simulink model "mech_interface_hyd_slidercrank"  (Simulink 7.1)
settings: Solver=ode15s  StartTime=0.0  StopTime=20  RelTol=1e-5
model workspace (MAT data in the model file):
  Lr = 0.5
  Lc = 0.288675134595
  sl_a = 0.5
  sl_b = 0.25
  sl_c = 0.25
  M_sl = 0.5
  I_sl = [0.0208333333333  0  0; 0  0.0520833333333  0; 0  0  0.0520833333333]
  rk_a = 0.5
  rk_b = 0.05
  rk_c = 0.05
  M_rk = 0.5
  I_rk = [0.000208333333333  0  0; 0  0.0105208333333  0; 0  0  0.0105208333333]
  cr_a = 0.288675
  cr_b = 0.05
  cr_c = 0.05
  M_cr = 5
  I_cr : num (value not decoded)
PostLoadFcn:
  | hws = get_param(bdroot, 'modelworkspace');
  | 
  | hws.assignin('sl_a', 0.5);
  | hws.assignin('sl_b', 0.25);
  | hws.assignin('sl_c', 0.25);
  | hws.assignin('M_sl', 0.5);
  | hws.evalin('I_sl = [1/3*M_sl*(sl_b^2 + sl_c^2) 0 0;   0 1/3*M_sl*(sl_a^2 + sl_c^2) 0;   0 0 1/3*M_sl*(sl_a^2 + sl_b^2)];')
  | 
  | hws.assignin('rk_a', 0.5);
  | hws.assignin('rk_b', 0.05);
  | hws.assignin('rk_c', 0.05);
  | hws.assignin('M_rk', 0.5);
  | hws.evalin('I_rk = [1/12*M_rk*(rk_b^2 + rk_c^2) 0 0;   0 1/12*M_rk*(rk_a^2 + rk_c^2) 0;   0 0 1/12*M_rk*(rk_a^2 + rk_b^2)];')
  | 
  | hws.assignin('cr_a', 0.288675);
  | hws.assignin('cr_b', 0.05);
  | hws.assignin('cr_c', 0.05);
  | hws.assignin('M_cr', 5);
  | hws.evalin('I_cr = [1/12*M_cr*(cr_b^2 + cr_c^2) 0 0;   0 1/12*M_cr*(cr_a^2 + cr_c^2) 0;   0 0 1/12*M_cr*(cr_a^2 + cr_b^2)];')
  | 
  | clear hws
undefined symbols (not defined in the file or in its folder): sigbuilder_block
libraries: mblibv1 x11, fl_lib x8, nesl_utility x3
Description:
  | Hydraulic - 3D Rotational Energy Conversion
  | 
  | The Rotational Hydraulic Actuator subsystem uses a Revolute-Rotational Interface block and Rotational Hydro-Mechanical Converter blocks to hydraulically actuate a revolute joint.
  | 
  | The hydraulic circuit is modeled in Simscape. The rest of the mechanism is modeled in SimMechanics.
settings Model: Creator=ksanthan  LastModifiedBy=batserve  ExtModeAutoUpdateStatusClock=off
settings SolverCC: SolverResetMethod=Robust
settings DataIOCC: SaveOutput=off  SignalLogging=off  SaveTime=off  OutputOption=SpecifiedOutputTimes  OutputTimes=[0:0.05:20]
settings DebuggingCC: AlgebraicLoopMsg=none  SignalResolutionControl=TryResolveAllWithWarning  SolverPrmCheckMsg=none
settings GRTTargetCC: TargetFcnLib=ansi_tfl_tmw_new.mat
settings SimMechanicsCC: VisOnUpdateDiagram=on  VisDuringSimulation=on

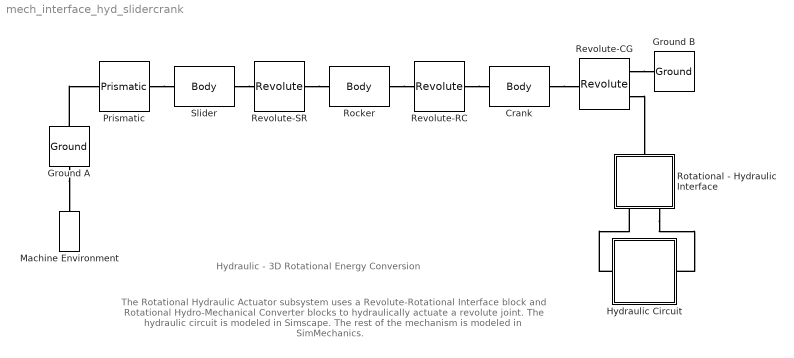
== system mech_interface_hyd_slidercrank ==
  note: Hydraulic - 3D Rotational Energy Conversion
  note: The Rotational Hydraulic Actuator subsystem uses a Revolute-Rotational Interface block and
      | Rotational Hydro-Mechanical Converter blocks to hydraulically actuate a revolute joint.
      |
      | The hydraulic circuit is modeled in Simscape.
      | The rest of the mechanism is modeled in SimMechanics.
  Crank : mblibv1/Bodies/Body  DialogController=MECH.DynMechDlgSource  PhysicalDomain=mechanical  SubClassName=Unknown  LeftPortType=workingframe  RightPortType=workingframe  LConnTagsString=CS1  RConnTagsString=CS2  DialogClass=MechanicalBodyBlock  Mass=M_cr  MassUnits=lbm  InertiaUnits=lbm*ft^2  Inertia=I_cr  Shape=Cylinder  ShapeDims=[1 1]  ShapeUnits=m  ShapeUse=false  Density=1  DensityUnits=kg/m^3  DensityUse=false  GraphicsMode=1  BodyColor=[0.5 0.5 0.5]  GraphicsObj=[]  AttachedToCS=1  CG=Left$CG$[cr_a 0 0]/2$CS1$CS1$ft$[0 0 0]$Euler X-Y-Z$deg$CS1$false  WorkingFrames=Left$CS1$[0 0 0]$Adjoining$Adjoining$ft$[0 0 -pi/2]$Euler X-Y-Z$rad$Adjoining$true#Right$CS2$[cr_a 0 0]$CS1$CS1$ft$[0 0 0]$Euler X-Y-Z$deg$CS1$true  CGPos=[cr_a 0 0]/2  CGRot=[0 0 0]  CS0Pos=[]  CS0Rot=[]  CS1Pos=[0 0 0]  CS1Rot=[0 0 -pi/2]  CS2Pos=[cr_a 0 0]  CS2Rot=[0 0 0]  CS3Pos=[]  CS3Rot=[]  CS4Pos=[]  CS4Rot=[]  CS5Pos=[]  CS5Rot=[]  CS6Pos=[]  CS6Rot=[]  CS7Pos=[]  CS7Rot=[]  CS8Pos=[]  CS8Rot=[]  CS9Pos=[]  CS9Rot=[]  CS10Pos=[]  CS10Rot=[]  CS11Pos=[]  CS11Rot=[]  CS12Pos=[]  CS12Rot=[]  CS13Pos=[]  CS13Rot=[]  CS14Pos=[]  CS14Rot=[]  CS15Pos=[]  CS15Rot=[]  CS16Pos=[]  CS16Rot=[]  CS17Pos=[]  CS17Rot=[]  CS18Pos=[]  CS18Rot=[]  CS19Pos=[]  CS19Rot=[]  CS20Pos=[]  CS20Rot=[]
  Ground A : mblibv1/Bodies/Ground  Orientation=up  DialogController=MECH.DynMechDlgSource  SystemSampleTime=-1  LeftPortType=env  RightPortType=workingframe  PhysicalDomain=Mechanical  DialogClass=GroundBlock  CoordPosition=[0 0 0]  CoordPositionUnits=m  StateVectorMgrId=-1  MachineId=[0 0]  ShowEnvPort=on
  Ground B : mblibv1/Bodies/Ground  Orientation=left  DialogController=MECH.DynMechDlgSource  SystemSampleTime=-1  LeftPortType=env  RightPortType=workingframe  PhysicalDomain=Mechanical  DialogClass=GroundBlock  CoordPosition=[Lr*cos(pi/6)+Lc*cos(pi/3)+1/24 0 0]  CoordPositionUnits=ft  StateVectorMgrId=-1  MachineId=[0 0]  ShowEnvPort=off
  Hydraulic Circuit : Subsystem
  Machine Environment : mblibv1/Bodies/Machine Environment  Tag=Factory ground  Orientation=up  DialogController=MECH.DialogSource  SystemSampleTime=-1  PortType=env  PhysicalDomain=Mechanical  DialogTemplateClass=MECH.MachineEnvironment  SyncWhenCopied=off  Gravity=[0 0 0]  GravityUnits=m/s^2  GravityAsSignal=off  Dimensionality=Auto-detect  AnalysisType=Forward dynamics  LinearAssemblyTolerance=1e-3  LinearAssemblyToleranceUnits=m  AngularAssemblyTolerance=1e-3  AngularAssemblyToleranceUnits=rad  ConstraintSolverType=Stabilizing  ConstraintRelTolerance=1e-4  ConstraintAbsTolerance=1e-4  UseRobustSingularityHandling=off  RedundancyAnalysisToleranceType=Automatically select tolerance  RedundancyAnalysisTolerance=1e-14  StatePerturbationType=Fixed  PerturbationSize=1e-5  VisualizeMachine=on
  Prismatic : mblibv1/Joints/Prismatic  DialogController=MECH.DynMechDlgSource  PhysicalDomain=mechanical  SubClassName=Unknown  LeftPortType=blob  RightPortType=blob  LConnTagsString=__newl0  RConnTagsString=__newr0  NumSAPorts=0  CutJoint=off  MarkAsCut=off  Primitives=prismatic  PrimitiveProps=P1$Base$[1 0 0]$prismatic  DialogClass=JointBlock  P1Axis=[1 0 0]
  Revolute-CG : mblibv1/Joints/Revolute  Orientation=left  DialogController=MECH.DynMechDlgSource  PhysicalDomain=mechanical  SubClassName=Unknown  LeftPortType=blob  RightPortType=blob  LConnTagsString=__newl0|SA1  RConnTagsString=__newr0  NumSAPorts=1  CutJoint=off  MarkAsCut=off  Primitives=prismatic  PrimitiveProps=R1$World$[0 0 1]$revolute  DialogClass=JointBlock  R1Axis=[0 0 1]
  Revolute-RC : mblibv1/Joints/Revolute  DialogController=MECH.DynMechDlgSource  PhysicalDomain=mechanical  SubClassName=Unknown  LeftPortType=blob  RightPortType=blob  LConnTagsString=__newl0  RConnTagsString=__newr0  NumSAPorts=0  CutJoint=off  MarkAsCut=off  Primitives=prismatic  PrimitiveProps=R1$Base$[0 0 1]$revolute  DialogClass=JointBlock  R1Axis=[0 0 1]
  Revolute-SR : mblibv1/Joints/Revolute  DialogController=MECH.DynMechDlgSource  PhysicalDomain=mechanical  SubClassName=Unknown  LeftPortType=blob  RightPortType=blob  LConnTagsString=__newl0  RConnTagsString=__newr0  NumSAPorts=0  CutJoint=off  MarkAsCut=off  Primitives=prismatic  PrimitiveProps=R1$Base$[0 0 1]$revolute  DialogClass=JointBlock  R1Axis=[0 0 1]
  Rocker : mblibv1/Bodies/Body  DialogController=MECH.DynMechDlgSource  PhysicalDomain=mechanical  SubClassName=Unknown  LeftPortType=workingframe  RightPortType=workingframe  LConnTagsString=CS1  RConnTagsString=CS2  DialogClass=MechanicalBodyBlock  Mass=M_rk  MassUnits=lbm  InertiaUnits=lbm*ft^2  Inertia=I_rk  Shape=Cylinder  ShapeDims=[1 1]  ShapeUnits=m  ShapeUse=false  Density=1  DensityUnits=kg/m^3  DensityUse=false  GraphicsMode=1  BodyColor=[0.5 0.5 0.5]  GraphicsObj=[]  AttachedToCS=1  CG=Left$CG$[rk_a 0 0]/2$CS1$CS1$ft$[0 0 0]$Euler X-Y-Z$deg$CS1$false  WorkingFrames=Left$CS1$[0 0 0]$Adjoining$Adjoining$ft$[0 0 pi/6]$Euler X-Y-Z$rad$Adjoining$true#Right$CS2$[rk_a 0 0]$CS1$CS1$ft$[0 0 0]$Euler X-Y-Z$deg$CS1$true  CGPos=[rk_a 0 0]/2  CGRot=[0 0 0]  CS0Pos=[]  CS0Rot=[]  CS1Pos=[0 0 0]  CS1Rot=[0 0 pi/6]  CS2Pos=[rk_a 0 0]  CS2Rot=[0 0 0]  CS3Pos=[]  CS3Rot=[]  CS4Pos=[]  CS4Rot=[]  CS5Pos=[]  CS5Rot=[]  CS6Pos=[]  CS6Rot=[]  CS7Pos=[]  CS7Rot=[]  CS8Pos=[]  CS8Rot=[]  CS9Pos=[]  CS9Rot=[]  CS10Pos=[]  CS10Rot=[]  CS11Pos=[]  CS11Rot=[]  CS12Pos=[]  CS12Rot=[]  CS13Pos=[]  CS13Rot=[]  CS14Pos=[]  CS14Rot=[]  CS15Pos=[]  CS15Rot=[]  CS16Pos=[]  CS16Rot=[]  CS17Pos=[]  CS17Rot=[]  CS18Pos=[]  CS18Rot=[]  CS19Pos=[]  CS19Rot=[]  CS20Pos=[]  CS20Rot=[]
  Rotational - Hydraulic Interface : Subsystem  Orientation=up
  Slider : mblibv1/Bodies/Body  DialogController=MECH.DynMechDlgSource  PhysicalDomain=mechanical  SubClassName=Unknown  LeftPortType=workingframe  RightPortType=workingframe  LConnTagsString=CS1  RConnTagsString=CG  DialogClass=MechanicalBodyBlock  Mass=M_sl  MassUnits=lbm  InertiaUnits=lbm*in^2  Inertia=I_sl  Shape=Cylinder  ShapeDims=[1 1]  ShapeUnits=m  ShapeUse=false  Density=1  DensityUnits=kg/m^3  DensityUse=false  GraphicsMode=1  BodyColor=[0.5 0.5 0.5]  GraphicsObj=[]  AttachedToCS=1  CG=Right$CG$[sl_a 0 0]$CS1$CS1$in$[0 0 0]$Euler X-Y-Z$deg$WORLD$true  WorkingFrames=Left$CS1$[0 0 0]$Adjoining$Adjoining$in$[0 0 0]$Euler X-Y-Z$deg$WORLD$true#Left$CS4$[0 sl_b 0]$CS1$CS1$in$[0 0 0]$Euler X-Y-Z$deg$WORLD$false#Right$CS6$[2*sl_a sl_b 0]$CS1$CS1$in$[0 0 0]$Euler X-Y-Z$deg$WORLD$false#Right$CS2$[2*sl_a 0 0]$CS1$CS1$in$[0 0 0]$Euler X-Y-Z$deg$WORLD$false#Right$CS5$[2*sl_a -sl_b 0]$CS1$CS1$in$[0 0 0]$Euler X-Y-Z$deg$WORLD$false#Left$CS3$[0 -sl_b 0]$CS1$CS1$in$[0 0 0]$Euler X-Y-Z$deg$WORLD$false  CGPos=[sl_a 0 0]  CGRot=[0 0 0]  CS0Pos=[]  CS0Rot=[]  CS1Pos=[0 0 0]  CS1Rot=[0 0 0]  CS2Pos=[2*sl_a 0 0]  CS2Rot=[0 0 0]  CS3Pos=[0 -sl_b 0]  CS3Rot=[0 0 0]  CS4Pos=[0 sl_b 0]  CS4Rot=[0 0 0]  CS5Pos=[2*sl_a -sl_b 0]  CS5Rot=[0 0 0]  CS6Pos=[2*sl_a sl_b 0]  CS6Rot=[0 0 0]  CS7Pos=[]  CS7Rot=[]  CS8Pos=[]  CS8Rot=[]  CS9Pos=[]  CS9Rot=[]  CS10Pos=[]  CS10Rot=[]  CS11Pos=[]  CS11Rot=[]  CS12Pos=[]  CS12Rot=[]  CS13Pos=[]  CS13Rot=[]  CS14Pos=[]  CS14Rot=[]  CS15Pos=[]  CS15Rot=[]  CS16Pos=[]  CS16Rot=[]  CS17Pos=[]  CS17Rot=[]  CS18Pos=[]  CS18Rot=[]  CS19Pos=[]  CS19Rot=[]  CS20Pos=[]  CS20Rot=[]
  connections:
  Slider/RConn1 -- Revolute-SR/LConn1
  Revolute-SR/RConn1 -- Rocker/LConn1
  Rocker/RConn1 -- Revolute-RC/LConn1
  Prismatic/RConn1 -- Slider/LConn1
  Ground A/RConn1 -- Prismatic/LConn1
  Ground A/LConn1 -- Machine Environment/RConn1
  Revolute-RC/RConn1 -- Crank/LConn1
  Hydraulic Circuit/LConn1 -- Rotational - Hydraulic Interface/LConn1
  Rotational - Hydraulic Interface/LConn2 -- Hydraulic Circuit/RConn1
  Revolute-CG/LConn1 -- Ground B/RConn1
  Crank/RConn1 -- Revolute-CG/RConn1
  Revolute-CG/LConn2 -- Rotational - Hydraulic Interface/RConn1

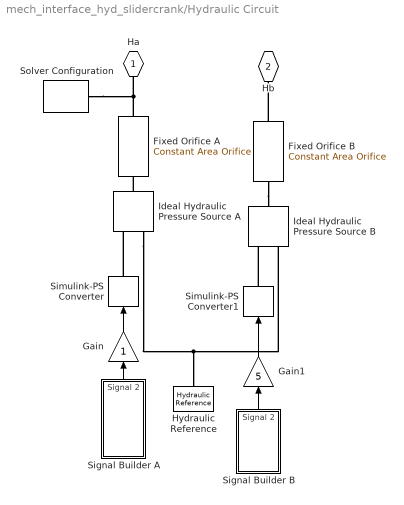
== system mech_interface_hyd_slidercrank/Hydraulic Circuit ==
  Fixed Orifice A : fl_lib/Hydraulic/Hydraulic Elements/Constant Area Orifice  Tag=Factory Generic  Orientation=up  DialogController=NetworkEngine.DynNeDlgSource  SystemSampleTime=-1  area=1e-04 m^2  C_d=0.7  Re_cr=12  flow_rate_Log=off  pr_drop_Log=off  power_Log=off  LocalVarNames=|flow_rate|pr_drop|Re|power  LocalVarDescs=|Flow rate through the orifice (m^3/s)|Pressure drop across the orifice (Pa)|Reynolds number|Power (W)  LocalVarLogging=[0 0 0 0]
  Fixed Orifice B : fl_lib/Hydraulic/Hydraulic Elements/Constant Area Orifice  Tag=Factory Generic  Orientation=up  DialogController=NetworkEngine.DynNeDlgSource  SystemSampleTime=-1  area=1e-04 m^2  C_d=0.7  Re_cr=12  flow_rate_Log=off  pr_drop_Log=off  power_Log=off  LocalVarNames=|flow_rate|pr_drop|Re|power  LocalVarDescs=|Flow rate through the orifice (m^3/s)|Pressure drop across the orifice (Pa)|Reynolds number|Power (W)  LocalVarLogging=[0 0 0 0]
  Gain : Gain  Orientation=up  ParameterDataType=sfix(16)  ParameterScaling=2^0  OutDataType=sfix(16)  OutScaling=2^0
  Gain1 : Gain  Orientation=up  Gain=5  ParameterDataType=sfix(16)  ParameterScaling=2^0  OutDataType=sfix(16)  OutScaling=2^0
  Hydraulic Reference : fl_lib/Hydraulic/Hydraulic Elements/Hydraulic Reference  Tag=Factory Generic  Orientation=down  DialogController=NetworkEngine.DynNeDlgSource  SystemSampleTime=-1  LocalVarLogging=[]
  Ideal Hydraulic Pressure Source A : fl_lib/Hydraulic/Hydraulic Sensors and Sources/Ideal Hydraulic Pressure Source  Tag=Factory Generic  Orientation=down  DialogController=NetworkEngine.DynNeDlgSource  SystemSampleTime=-1  flow_rate_Log=off  pr_differential_Log=off  power_Log=off  LocalVarNames=|flow_rate|pr_differential|power  LocalVarDescs=|Flow rate through the source (m^3/s)|Pressure differential across the source (Pa)|Source power (W)  LocalVarLogging=[0 0 0]
  Ideal Hydraulic Pressure Source B : fl_lib/Hydraulic/Hydraulic Sensors and Sources/Ideal Hydraulic Pressure Source  Tag=Factory Generic  Orientation=down  DialogController=NetworkEngine.DynNeDlgSource  SystemSampleTime=-1  flow_rate_Log=off  pr_differential_Log=off  power_Log=off  LocalVarNames=|flow_rate|pr_differential|power  LocalVarDescs=|Flow rate through the source (m^3/s)|Pressure differential across the source (Pa)|Source power (W)  LocalVarLogging=[0 0 0]
  Signal Builder A : Subsystem  Tag=STV Subsys  Orientation=up  LoadFcn=sigbuilder_block('load');  StartFcn=sigbuilder_block('start');  StopFcn=sigbuilder_block('stop');  ClipboardFcn=sigbuilder_block('clipboard');  mask(Sigbuilder block){}
      mask help: Sigbuilder GUI
      mask init:
      | if ~strcmp(get_param(bdroot(gcbh),'SimulationStatus'),'stopped') tuvar = sigbuilder_block('maskInit'); end
      settings: CopyFcn=sigbuilder_block('copy');  DeleteFcn=sigbuilder_block('delete');  ModelCloseFcn=sigbuilder_block('modelClose');  PreSaveFcn=sigbuilder_block('preSave');  NameChangeFcn=sigbuilder_block('namechange');  OpenFcn=sigbuilder_block('open',[160.5 256.5 550.5 399.75 ]);  CloseFcn=sigbuilder_block('close');
      mask Display: plot(0,0,100,100,[10,10,40,40,10],[80,20,20,80,80],[40,10],[50,50], [40,27,10],[65,72,56],[40,25,25,10],[28,28,43,43]);
  Signal Builder B : Subsystem  Tag=STV Subsys  Orientation=up  LoadFcn=sigbuilder_block('load');  StartFcn=sigbuilder_block('start');  StopFcn=sigbuilder_block('stop');  ClipboardFcn=sigbuilder_block('clipboard');  mask(Sigbuilder block){}
      mask help: Sigbuilder GUI
      mask init:
      | if ~strcmp(get_param(bdroot(gcbh),'SimulationStatus'),'stopped') tuvar = sigbuilder_block('maskInit'); end
      settings: CopyFcn=sigbuilder_block('copy');  DeleteFcn=sigbuilder_block('delete');  ModelCloseFcn=sigbuilder_block('modelClose');  PreSaveFcn=sigbuilder_block('preSave');  NameChangeFcn=sigbuilder_block('namechange');  OpenFcn=sigbuilder_block('open',[405 251.25 550.5 399.75 ]);  CloseFcn=sigbuilder_block('close');
      mask Display: plot(0,0,100,100,[10,10,40,40,10],[80,20,20,80,80],[40,10],[50,50], [40,27,10],[65,72,56],[40,25,25,10],[28,28,43,43]);
  Simulink-PS Converter : nesl_utility/Simulink-PS Converter  Orientation=up  DialogController=NetworkEngine.DynNeUtilDlgSource  SystemSampleTime=-1  PhysicalDomain=network_engine_domain  LeftPortType=input  RightPortType=output  SubClassName=ps_input  Unit=bar  AffineConversion=off
  Simulink-PS Converter1 : nesl_utility/Simulink-PS Converter  Orientation=up  DialogController=NetworkEngine.DynNeUtilDlgSource  SystemSampleTime=-1  PhysicalDomain=network_engine_domain  LeftPortType=input  RightPortType=output  SubClassName=ps_input  Unit=bar  AffineConversion=off
  Solver Configuration : nesl_utility/Solver Configuration  DialogController=NetworkEngine.DynNeUtilDlgSource  SystemSampleTime=-1  PhysicalDomain=network_engine_domain  LeftPortType=input  RightPortType=generic  SubClassName=solver  Accelerate=off  Profile=off  ResidualTolerance=1e-9  MaxNonlinIter=12  MaxModeIter=2  DoFixedCost=off  DoDC=off  LinearAlgebra=Sparse
  Ha : PMIOPort  Orientation=down  Port=1  Side=Left
  Hb : PMIOPort  Orientation=down  Port=2  Side=Right
  wires:
  Gain/1 -> Simulink-PS Converter/1
  Signal Builder A/1(Signal 2) -> Gain/1
  Gain1/1 -> Simulink-PS Converter1/1
  Signal Builder B/1(Signal 2) -> Gain1/1
  connections:
  Fixed Orifice B/RConn1 -- Hb/RConn1
  Simulink-PS Converter/RConn1 -- Ideal Hydraulic Pressure Source A/RConn1
  Ideal Hydraulic Pressure Source A/LConn1 -- Fixed Orifice A/LConn1
  Fixed Orifice B/LConn1 -- Ideal Hydraulic Pressure Source B/LConn1
  Simulink-PS Converter1/RConn1 -- Ideal Hydraulic Pressure Source B/RConn1
  Ideal Hydraulic Pressure Source A/RConn2 -- Ideal Hydraulic Pressure Source B/RConn2 -- Hydraulic Reference/LConn1
  Fixed Orifice A/RConn1 -- Ha/RConn1 -- Solver Configuration/RConn1

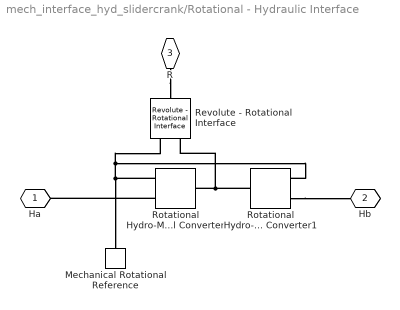
== system mech_interface_hyd_slidercrank/Rotational - Hydraulic Interface ==
  Mechanical Rotational Reference : fl_lib/Mechanical/Rotational Elements/Mechanical Rotational Reference  Orientation=down  DialogController=NetworkEngine.DynNeDlgSource  SystemSampleTime=-1  LocalVarLogging=[]
  Revolute - Rotational Interface : mblibv1/Interface  Elements/Revolute - Rotational Interface  Orientation=up  DialogController=MECH.DynMechDlgSource  SystemSampleTime=-1  DialogClass=RevoluteRotationalInterface  Primitive=R1
  Rotational Hydro-Mechanical Converter : fl_lib/Hydraulic/Hydraulic Elements/Rotational Hydro-Mechanical Converter  DialogController=NetworkEngine.DynNeDlgSource  SystemSampleTime=-1  D=1.2e-04 m^3/rad  or=1  flow_rate_Log=off  pressure_Log=off  torque_Log=off  ang_velocity_Log=off  power_Log=off  LocalVarNames=|flow_rate|pressure|torque|ang_velocity|power  LocalVarDescs=|Flow rate into the chamber (m^3/s)|Pressure at the inlet (Pa)|Output torque (N*m)|Shaft angular velocity (rad/s)|Power (W)  LocalVarLogging=[0 0 0 0 0]
  Rotational Hydro-Mechanical Converter1 : fl_lib/Hydraulic/Hydraulic Elements/Rotational Hydro-Mechanical Converter  Orientation=left  DialogController=NetworkEngine.DynNeDlgSource  SystemSampleTime=-1  D=1.2e-04 m^3/rad  or=2  flow_rate_Log=off  pressure_Log=off  torque_Log=off  ang_velocity_Log=off  power_Log=off  LocalVarNames=|flow_rate|pressure|torque|ang_velocity|power  LocalVarDescs=|Flow rate into the chamber (m^3/s)|Pressure at the inlet (Pa)|Output torque (N*m)|Shaft angular velocity (rad/s)|Power (W)  LocalVarLogging=[0 0 0 0 0]
  Ha : PMIOPort  Tag=PMCPort  Port=1  Side=Left
  Hb : PMIOPort  Tag=PMCPort  Orientation=left  Port=2  Side=Left
  R : PMIOPort  Tag=PMCPort  Orientation=down  Port=3  Side=Right
  connections:
  R/RConn1 -- Revolute - Rotational Interface/RConn1
  Revolute - Rotational Interface/LConn1 -- Rotational Hydro-Mechanical Converter/LConn1 -- Mechanical Rotational Reference/LConn1 -- Rotational Hydro-Mechanical Converter1/LConn1
  Rotational Hydro-Mechanical Converter/LConn2 -- Ha/RConn1
  Rotational Hydro-Mechanical Converter1/LConn2 -- Hb/RConn1
  Revolute - Rotational Interface/LConn2 -- Rotational Hydro-Mechanical Converter1/RConn1 -- Rotational Hydro-Mechanical Converter/RConn1

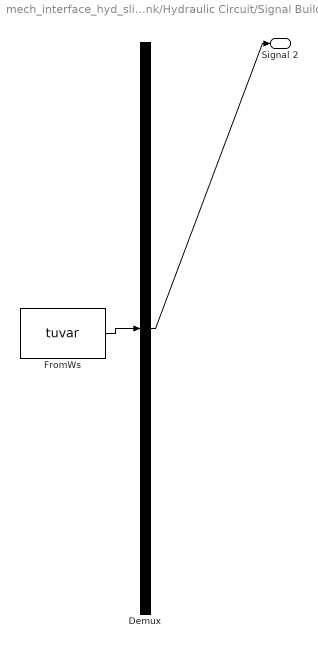
== system mech_interface_hyd_slidercrank/Hydraulic Circuit/Signal Builder A ==
  Demux : Demux  Tag=STV Demux  Outputs=1
  FromWs : FromWorkspace  Tag=STV FromWs  VariableName=tuvar  SampleTime=0  SigBuilderData=DataTag3  VnvData=DataTag4
      SigBuilderData=|
      | channels.label = 'Signal 2'
      | channels.allXData = {[0 0.98 1.96 2.96 4 6 12 13 13 14 15 15.95 20]}
      | channels.allYData = {[0 1.005 1 0.995 0.045 0.045 0.045 0.005 0 0 0.005 0.005 0.005]}
      | common.afterFinalStr = 'Extrapolate'
      | common.sampleTime = 0
      | dataSet.timeRange = [0 20]
      | dataSet.name = 'Group 1'
  Signal 2 : Outport  Tag=STV Outport  OutDataType=sfix(16)  OutScaling=2^0
  wires:
  Demux/1 -> Signal 2/1
  FromWs/1 -> Demux/1

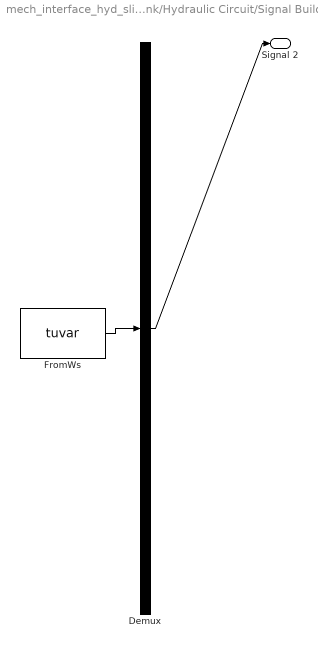
== system mech_interface_hyd_slidercrank/Hydraulic Circuit/Signal Builder B ==
  Demux : Demux  Tag=STV Demux  Outputs=1
  FromWs : FromWorkspace  Tag=STV FromWs  VariableName=tuvar  SampleTime=0  SigBuilderData=DataTag5  VnvData=DataTag6
      SigBuilderData=|
      | channels.label = 'Signal 2'
      | channels.allXData = {[0 0.98 1.96 2.96 4 6 12 13 14 15 15 15.95 15.95 20]}
      | channels.allYData = {[0 0 0.005 0.005 0.005 0 0.005 1 1 1.005 1 0.03 0.02 0.02]}
      | common.afterFinalStr = 'Extrapolate'
      | common.sampleTime = 0
      | dataSet.timeRange = [0 20]
      | dataSet.name = 'Group 1'
  Signal 2 : Outport  Tag=STV Outport  OutDataType=sfix(16)  OutScaling=2^0
  wires:
  FromWs/1 -> Demux/1
  Demux/1 -> Signal 2/1
